simulink library "Library_SignalGeneration"  (R2017b)
settings: Solver=ode45  StartTime=0.0  StopTime=10.0  RelTol=1e-3  EnableMultiTasking=on
undefined symbols (not defined in the file): DiscIntNeverNeededParam, Fif, Fs, jsin, Ts
libraries: simulink x8, Library_SignalGeneration x5, simulink_need_slupdate x1
settings Model: Creator=Keith  LastModifiedBy=sawmilkd
settings DataIOCC: LimitDataPoints=on
settings OptimizationCC: LifeSpan=inf
settings DebuggingCC: AllowSymbolicDim=off  SFUnexpectedBacktrackingDiag=warning  SFNoUnconditionalDefaultTransitionDiag=warning  SFExecutionAtInitializationDiag=none
settings CodeAppCC: StateflowObjectComments=on
settings GRTTargetCC: TargetLangStandard=C89/C90 (ANSI)  GeneratePreprocessorConditionals=Disable all
settings ConfigComp: CovMetricSettings=dw  CovHtmlReporting=on  CovSaveCumulativeToWorkspaceVar=on  CovSaveSingleToWorkspaceVar=on  CovExternalEMLEnable=off

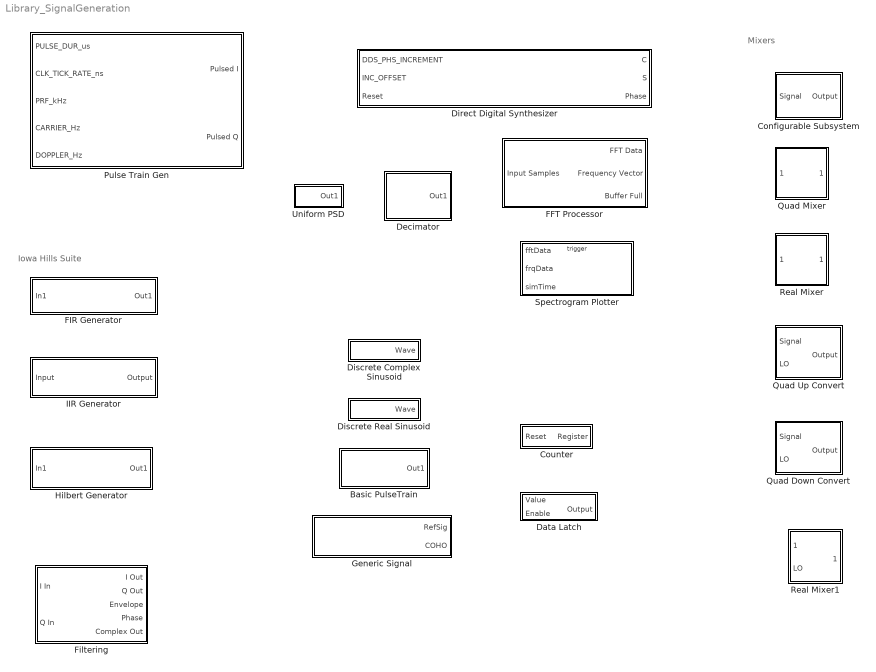
== system Library_SignalGeneration ==
  note: Iowa Hills Suite
  note: Mixers
  Basic PulseTrain : Subsystem  mask{Fs=245.76e6, PRF=633000, Fc=50e6, PD=0.6}
      mask prompts: Fs "Clock Rate"; PRF "PRF (Hz)"; Fc "Carrier (Hz)"; PD "Pulsewidth (us)"
      mask init:
      | iprf = floor(Fs/PRF)
      | ipd = floor(Fs*PD*1e-6)
      mask DialogControl DescTextVar Prompt: Generates clock-matched pulsetrain. This is the simplest form of pulsetrain generation.
      mask Display:
      | port_label('output',1,'')
      | disp([ ...
      |     'PRF: ' num2str(PRF) ' Hz\n' ...
      |     'PD: ' num2str(PD) ' us\n' ...
      |     'Fc: ' num2str(Fc/1e6) ' MHz' ...
      |     ]);
  Configurable Subsystem : Subsystem  BlockChoice=Quad Mixer
      settings: TemplateBlock=self  MemberBlocks=Quad Mixer,Real Mixer
  Counter : Subsystem  mask{nBits=0}
      mask prompts: nBits "Bits"
      mask Display:
      | nb = str2num(get_param(gcb,'nBits'));
      | if(nb == 0)
      |     disp(['CTR']);
      | 
      | else
      |     disp(['CTR' num2str(nb,'%d')]);
      | end
      | port_label('input',1,'R');
      | port_label('output',1,'O');
  Data Latch : Subsystem
  Decimator : Subsystem  mask{parentFs=Fs, decFac=2}
      mask prompts: parentFs "Parent Sample Rate"; decFac "Decimation Factor"
      mask DialogControl Control2 Prompt: Minimum Decimation is 2
      mask Display:
      | FD=parentFs/decFac;
      | str = 'Hz';
      | if(FD > 1e6)
      |     FD = FD/1e6;
      |     str = 'MHz';
      | elseif(FD > 1e3);
      |     FD = FD/1e3;
      |     str = 'kHz';
      | end
      | disp([num2str(decFac) ':1\nFD = ' num2str(FD) str])
  Direct Digital Synthesizer : Subsystem  mask{Fs=245.76e6, Nbits=28, useFreqInput=on}
      mask prompts: Fs "Clock Speed (Hz)"; Nbits "Bits"; useFreqInput "Frequency Based Input"
      mask DialogControl Control2 Prompt: This block can be configured to accept either integer phase increment and offsets or frequency (Hz) as an input
      mask Display:
      | if(useFreqInput)
      |     port_label('input',1,'F_Hz');
      |     port_label('input',2,'FO_Hz');
      | else
      |     port_label('input',1,'DDS_PHASE_INCREMENT')
      |     port_label('input',2,'DDS_PHASE_INC_OFFSET');
      | end
      | port_label('input',3,'Rst');
      | 
      | port_label('output',1,'Cos');
      | port_label('output',2,'Sin');
      | port_label('output',3,'Phase');
      | 
      | fprintf('Fs = %6.2fMHz\nBits = %d',Fs/1e6,Nbits);
  Discrete Complex Sinusoid : Subsystem  mask{initPhase=0*pi/180, freqHz=1e6-2000}
      mask prompts: initPhase "Starting Phase (rad)"; freqHz "Frequency (Hz)"
      settings: AttributesFormatString=|
      | Frequency: %<freqHz>
      | Starting Phase: %<initPhase>
  Discrete Real Sinusoid : Subsystem  mask{freqHz=5e6}
      mask prompts: freqHz "Frequency (Hz)"
      settings: AttributesFormatString=Frequency: %<freqHz>
  FFT Processor : Subsystem  mask{BUFFSIZE=2^10, FFTSIZE=2^10, FOUTRNG=[15 30]*1e6, OVLP_PRCNT=95, Fs=Fs, FSCALE=1e-6}
      mask prompts: BUFFSIZE "Buffer Size"; FFTSIZE "FFT Size"; FOUTRNG "Output Freq Range"; OVLP_PRCNT "% Overlap"; Fs "Input Rate"; FSCALE "Frequency Output Scale Factor"
      mask init:
      | %if(BUFFSIZE > FFTSIZE)
      | %    errordlg(['Buffer size (' num2str(BUFFSIZE) ') cannot exceed FFT size (' num2str(FFTSIZE) ').']);
      | %    BUFFSIZE = FFTSIZE;
      | %end
      | OVLP_FRAMES = floor((1-OVLP_PRCNT/100) * BUFFSIZE);
      | disp(['Overlap Frames: ' num2str(OVLP_FRAMES)]);
      | 
      | RateOut = Fs / BUFFSIZE;
      | DF = Fs / FFTSIZE;
      | 
      | 
      | 
      | if(isempty(FOUTRNG))
      |     FFTIDX = 1:FFTSIZE;
      | else
      |     spn = floor((FOUTRNG./Fs)*FFTSIZE);
      |     FFTIDX = spn(1):spn(2);
      | end
      | 
      | FFT_SIZE_OUT = length(FFTIDX);
      mask DialogControl Control2 Prompt: Buffer Size determines how many samples are accumulated before computing the FFT
      mask DialogControl Control3 Prompt: FFT Size determines how many samples (actual + zero padded) are passed to the FFT algorithm.
      mask DialogControl Control4 Prompt: Select the [fmin fmax] desired out of the FFT processor, or leave as [] to get the full spectrum.
      mask DialogControl Container3 Prompt: Information
      mask Display:
      | TimeOut = 1/RateOut;
      | if( TimeOut < 1.0e-3 )
      |     sf = 1.0e6;
      |     str = 'us';
      | elseif( TimeOut < 1.0e-0 )
      |     sf = 1000;
      |     str = 'ms';
      | else
      |     sf = 1;
      |     str = 's';
      | end
      | 
      | disp(['FO: ' num2str(RateOut) ' Hz'...
      |     '\nDF: ' num2str(DF) ' Hz' ...
      |     '\nDT: ' num2str(sf*TimeOut) str]);
      | port_label('input',1,'In');
      | port_label('output',1,'FFT');
      | port_label('output',2,'FRQ');
      | port_label('output',3,'FULL');
  FIR Generator : Subsystem  mask{ihFilename=<not specified>, ihFilenameResolved=<not specified>, fileIsVar=off, shiftEnable=off, shiftFactor=.3}
      mask prompts: ihFilename "Iowa Hills FIR Coefficient File"; fileIsVar "Filename above is a variable"; shiftEnable "Enable Quadrature Shifting"; shiftFactor "Shift Ratio (fraction of Fs)"
      mask init:
      | % Note: You can "access" dialog data directly, but to change
      | %       it, use the set_param command.
      | 
      | % Manage the dialog data. It can be:
      | % 1 - A filename, or 2 - A variable that evaluates to 
      | %     a filename.
      | 
      | % first, check for iowa hills code
      | s = which('FirFilterC');
      | if(isempty(s))
      |     errordlg('Iowa Hills not found in search path!','Iowa Hills Error');
      |     return;
      | end
      | 
      | 
      | instr = [];
      | if(~fileIsVar && ~strcmpi(ihFilename,'<not specified>'))
      |     instr = ihFilename;
      | elseif(fileIsVar && ~strcmpi(ihFilename,'<not specified>'))
      |     try
      |         instr = eval(ihFilename);
      |     catch
      |         instr = evalin('base',ihFilename);
      |     end
      | end
      | 
      | % Create MATLAB instance
      | if(~isempty(instr))
      |     set_param(gcb,'ihFilenameResolved',instr);
      |     
      |     if(~exist(instr,'file'))
      |         errordlg(['Could not locate file ' instr],'File Error');
      |         return;
      |     end
      |     
      |     local_instance = FirFilterC(instr);
      |     
      |     if(shiftEnable == 1)
      |         local_instance.shiftFir(shiftFactor,1);    
      |     end
      |     
      |     this_model = gcb;
      |     tgt_model = [this_model '/Discrete FIR Filter'];
      |     set_param(tgt_model,'Coefficients',['[' num2str(local_instance.tapgains.','%18.14f') ']']);
      | else
      |     set_param(gcb,'ihFilenameResolved','<not specified>');
      | end
      settings: AttributesFormatString=|
      | FIR File:  %<ihFilenameResolved>
      | Quad Shift: %<shiftEnable>,%<shiftFactor>
      mask DialogControl DescTextVar Prompt: Use the Iowa Hills Tools to develop the filter. You may either type the filename below, or store the filename as a variable and check the box below. In that case, enter the variable name in the field.
      mask DialogControl Control2 Prompt: The filter definition above may be shifted in frequency via quadrature shifting. This will create complex weights, but enables full spectrum IQ filtering
      mask Display:
      | s = get_param(gcb,'ihFilename');
      | if(strcmpi(s,'<not specified>'))
      |     fprintf('Iowa Hills FIR Filter\n %s',s);
      | else
      |     NFFT = 8192;
      |     xi = 0:NFFT-1;
      |     yi = str2num(get_param([gcb '/Discrete FIR Filter'],'Coefficients'));
      |     color('red');
      |     plot(xi,20*log10(abs(fft(yi,NFFT))));
      | end
  Filtering : Subsystem  mask{ihFirFile=BPF_50MHZ_245p76MGZ.txt}
      mask prompts: ihFirFile "Iowa Hills FIR Filter File"
      settings: AttributesFormatString=File: %<ihFirFile>
  Generic Signal : Subsystem  mask{fPoints=[0 0]*1e6 + Fif, dPoints=[20 24]*1e3, tPoints=[0 40*24e-3], isPulsed=on, PRF=600e3, PD=.5e-6, FS=Fs}
      mask prompts: fPoints "COHO Points"; dPoints "Doppler Points"; tPoints "Time Points"; isPulsed "Is Pulsed"; PD "Pulsewidth"
      mask init:
      | if(isPulsed)
      |     ipri = floor(FS/PRF);
      |     ipd = floor(FS * PD);
      | else
      |     ipri = 1;
      |     ipd = 1;
      | end
      | 
      | %disp([ipri ipd])
      mask Callback isPulsed:
      | if(strcmp('on',get_param(gcb,'isPulsed')))
      |     me = get_param(gcb,'MaskEnables');
      |     me{5} = 'on';
      |     me{6} = 'on';
      |     me{7} = 'on';
      | else
      |     me = get_param(gcb,'MaskEnables');
      |     me{5} = 'off';
      |     me{6} = 'off';
      |     me{7} = 'off';
      | end
      | set_param(gcb,'MaskEnables',me);
      mask DialogControl DescTextVar Prompt: Generates a reference quadrature signal with frequency properties specified over time
      mask DialogControl Control2 Prompt: COHO is Output CW, Doppler is not
      mask Display:
      | port_label('output',1,'SIG')
      | port_label('output',2,'COHO')
      | 
      | if(fPoints(1) > 1e6)
      |     fsc = 1e-6;
      |     fstr = 'MHz';
      | elseif(fPoints(1) > 1e3)
      |     fsc = 1e-3;
      |     fstr = 'kHz';
      | else
      |     fsc = 1.0;
      |     fstr = 'Hz';
      | end
      | 
      | if(PRF > 1e3)
      |     prfsc = 1e-3;
      |     prfstr = 'kHz';
      | else
      |     prfsc = 1.0;
      |     prfstr = 'Hz';
      | end
      | 
      | if(PD > 1e-3)
      |     pdsc = 1e3;
      |     pdstr = 'ms';
      | elseif(PD > 1e-6)
      |     pdsc = 1e6;
      |     pdstr = 'us';
      | elseif(PD > 1e-9)
      |     pdsc = 1e9;
      |     pdstr = 'ns';
      | end
      | 
      | 
      | if(isPulsed)
      |     text(0.15,.5,sprintf('F1=%4.2f%s\nPRF=%4.2f%s\nPW=%4.2f%s', ...
      |         fsc * fPoints(1),fstr,prfsc*PRF,prfstr,pdsc*PD,pdstr))
      | else
      |     text(0.15,.5,sprintf('F1=%4.2eHz\n\n',fPoints(1)))
      | end
  Hilbert Generator : Subsystem  mask{ihFilename=<not specified>, fileIsVar=off, ihFilenameResolved=<not specified>}
      mask prompts: ihFilename "Iowa Hills Hilbert Coefficient File"; fileIsVar "Filename above is a variable"
      mask init:
      | % Manage the dialog data. It can be:
      | % 1 - A filename, or 2 - A variable that evaluates to 
      | %     a filename.
      | instr = [];
      | if(~fileIsVar && ~strcmpi(ihFilename,'<not specified>'))
      |     instr = ihFilename;
      | elseif(fileIsVar && ~strcmpi(ihFilename,'<not specified>'))
      |     try
      |         instr = eval(ihFilename);
      |     catch
      |         instr = evalin('base',ihFilename);
      |     end
      | end
      | 
      | % Create MATLAB instance
      | if(~isempty(instr))
      |     set_param(gcb,'ihFilenameResolved',instr);
      |     local_instance = HilbertFilter(instr);
      |     this_model = gcb;
      |     tgt_model = [this_model '/Discrete FIR FilterI'];
      |     set_param(tgt_model,'Coefficients',['[' num2str(local_instance.iChanFIR.tapgains.','%18.14f') ']']);
      |     tgt_model = [this_model '/Discrete FIR FilterQ'];
      |     set_param(tgt_model,'Coefficients',['[' num2str(local_instance.qChanFIR.tapgains.','%18.14f') ']']);
      | else
      |     set_param(gcb,'ihFilenameResolved','<not specified>');
      | end
      settings: AttributesFormatString="Hilbert File:  %<ihFilenameResolved>"
      mask DialogControl DescTextVar Prompt: Use the Iowa Hills Tools to develop the filter. You may either type the filename below, or store the filename as a variable and check the box below. In that case, enter the variable name in the field.
      mask Display:
      | s = get_param(gcb,'ihFilename');
      | if(strcmpi(s,'<not specified>'))
      |     fprintf('Iowa Hills Hilbert Filter\n %s',s);
      | else
      |     NFFT = 8192;
      |     xi = 0:NFFT-1;
      |     yi = str2num(get_param([gcb '/Discrete FIR FilterQ'],'Coefficients'));
      |     color('red');
      |     plot(xi,20*log10(abs(fft(yi,NFFT))));
      | end
  IIR Generator : Subsystem  mask{ihFilename=<not specified>, shiftEnable=off, shiftFactor=0.5, bodeplt=0}
      mask prompts: ihFilename "Iowa Hills IIR Coefficient File"; shiftEnable "Enable Quadrature Shifting"; shiftFactor "Shift Ratio (fraction of Fs)"
      mask init:
      | %disp('Running IIR Init Mask Function')
      | 
      | % attempt to build IIR stages block via program
      | 
      | % first, read the file from MATLAB IH code
      | %disp([' Input Name: ' ihFilename]);
      | 
      | if(strcmp(ihFilename,'<not specified>'))
      |     return;
      | end
      | 
      | iir_file = ihFilename;
      | 
      | if(~exist(iir_file,'file'))
      |     errordlg(['Could not locate file ' iir_file],'File Error');
      |     return;
      | end
      | 
      | % Read in data
      | %local_instance = biquad_stages(0);
      | s = which('biquad_stages');
      | if(~isempty(s))
      |     local_instance = biquad_stages(iir_file);
      | else
      |     errordlg('Iowa Hills not found in search path!','Iowa Hills Error');
      |     return;
      | end
      | if(shiftEnable == 1)
      |    local_instance = local_instance.shiftStages(shiftFactor,1);    
      | end
      | npts=8192;
      | da = 2*pi*(0:npts)./npts;
      | z  = exp(1i*da);
      | bodeplt = 20*log10(abs(evalFilterZ(local_instance,z)));
      | %[a0,a1,a2,b0,b1,b2] = read_iowa_hills(iir_file);
      | 
      | src_model = gcb;
      | %disp([' Source model: ' src_model]);
      | 
      | % Prep model for building
      | h_lines = get_param(src_model,'Lines');
      | if(~isempty(h_lines))
      |     delete(h_lines(:).Handle);
      | end
      | 
      | h_blocks = get_param(src_model,'Blocks');
      | 
      | for k = 1 : length(h_blocks)
      |     if(strfind(h_blocks{k},'Stage'))
      |         %disp(['  Deleting existing block ' h_blocks{k}]);
      |         delete_block([src_model '/' h_blocks{k}])
      |     end
      | end
      | 
      | 
      | % spacing parameters
      | p_xstart = 70;
      | p_xoffset = 80;
      | 
      | nStages = local_instance.nstages;
      | %return;
      | %open_system(src_model);
      | 
      | dest_block_in = [src_model '/Input'];
      | %add_block( ...
      | %    'simulink/Sources/In1', ...
      | %    dest_block_in);
      | set_param(dest_block_in,'Position', ...
      |     [0+p_xstart 38 0+30+p_xstart 52]);
      | 
      | 
      | for istage = 1 :nStages
      |     dest_block = [src_model '/Stage ' num2str(istage-1)];
      |     add_block( ...
      |         'simulink/Discrete/Discrete Filter', ...
      |         dest_block);
      |     
      |     % NOTE: Position is topleft x,y, botright x,y
      |     xoffset = p_xoffset*(istage);
      |     xstart = p_xstart;
      |     set_param(dest_block,'Position',[xstart+xoffset 25 xstart+50+xoffset 60]);
      |     
      |     % set the connection to blocks
      |     if(istage == 1)
      |         add_line(src_model,'Input/1','Stage 0/1');
      |     else
      |         add_line(src_model, ...
      |             ['Stage ' num2str(istage-2) '/1'], ...
      |             ['Stage ' num2str(istage-1) '/1']);
      |     end
      |     
      |     % evaluate shifting
      |     %disp(shiftEnable)
      | %     if(shiftEnable == 1)
      | %          k = 1; sc1 = exp(1i*2*pi*shiftFactor*k);
      | %          k = 2; sc2 = exp(1i*2*pi*shiftFactor*k);
      | %     else
      | %         sc1 = 1;
      | %         sc2 = 1;
      | %     end
      |     
      |     
      |     % set the coefficients
      |     %str = ['[' num2str([a0(istage) sc1*a1(istage) sc2*a2(istage)],'%18.14f ') ']'];
      |     str = ['[' num2str(local_instance.biquads(istage).A,'%18.14f') ']'];
      |     set_param(dest_block,'Denominator',str);
      |     %str = ['[' num2str([b0(istage) sc1*b1(istage) sc2*b2(istage)],'%18.14f ') ']'];
      |     str = ['[' num2str(local_instance.biquads(istage).B,'%18.14f') ']'];
      |     set_param(dest_block,'Numerator',str);
      |     set_param(dest_block,'SampleTime','-1');
      |     
      | end
      | 
      | dest_block_out = [src_model '/Output'];
      | %add_block( ...
      | %    'simulink/Sinks/Out1', ...
      | %    dest_block_out);
      | xoffset = p_xoffset*(istage+1);
      | set_param(dest_block_out,'Position', ...
      |     [0+p_xstart+xoffset 38 0+30+p_xstart+xoffset 52]);
      | 
      | add_line(src_model, ...
      |         ['Stage ' num2str(istage-1) '/1'], ...
      |         ['Output/1']);
      settings: AttributesFormatString=|
      | IIR File:  %<ihFilename>
      | Quad Shift: %<shiftEnable>,%<shiftFactor>
      mask DialogControl Control2 Prompt: The filter definition above may be shifted in frequency via quadrature shifting. This will create complex weights, but enables full spectrum IQ filtering
      mask Display:
      | s = get_param(gcb,'ihFilename');
      | if(strcmpi(s,'<not specified>'))
      |     fprintf('Iowa Hills IIR Filter\n %s',s);
      | else
      |     plot(bodeplt);
      | end
  Pulse Train Gen : Subsystem
  Quad Down Convert : Subsystem
      mask Display: image('mixer_3port.png');
  Quad Mixer : Subsystem  mask{loFrequencyHz=-4e6}
      mask prompts: loFrequencyHz "LO Frequency (Hz)"
      settings: AttributesFormatString=LO: %<loFrequencyHz>
      mask DialogControl DescTextVar Prompt: This block will take a complex input and either upconvert (+) or downconvert (-) by the mixing with a complex specified LO (below)
      mask Display:
      | image('mixer2.png');
      | %port_label('output', 1, 'O')
      | %port_label('input', 1, 'I')
  Quad Up Convert : Subsystem
      mask Display: image('mixer_3port.png');
  Real Mixer : Subsystem  mask{loFrequencyHz=-4e6}
      mask prompts: loFrequencyHz "LO Frequency (Hz)"
      settings: AttributesFormatString=LO: %<loFrequencyHz>
      mask DialogControl DescTextVar Prompt: This block will take a complex input and either upconvert (+) or downconvert (-) by the mixing with a complex specified LO (below)
      mask Display:
      | image('mixer2.png');
      | %port_label('output', 1, 'O')
      | %port_label('input', 1, 'I')
  Real Mixer1 : Subsystem  mask{loFrequencyHz=-4e6}
      mask prompts: loFrequencyHz "LO Frequency (Hz)"
      settings: AttributesFormatString=LO: %<loFrequencyHz>
      mask DialogControl DescTextVar Prompt: This block will take a complex input and either upconvert (+) or downconvert (-) by the mixing with a complex specified LO (below)
      mask Display:
      | %image('mixer2.png');
      | port_label('output', 1, 'IF')
      | port_label('input', 2, 'RF')
      | port_label('input', 1, 'LO')
  Spectrogram Plotter : MATLAB Function  StopFcn=disp('done')  TreatAsAtomicUnit=on  mask{nRows=64, complexFFT=on, Fs=1000, Zo=50, cMin=-60, cMax=10}
      mask prompts: nRows "Rows in Image"; complexFFT "Quadrature Data? (Use Fs vs Fs/2)"; Fs "Sample Rate (Hz)"; Zo "Characteristic Impedance (Ohms)"; cMin "Minimum Power Scale"; cMax "Maximum Power Scale"
      settings: AttributesFormatString=|
      | Fs=%<Fs> | Zo=%<Zo>
      | Displays %<nRows> Rows
  Uniform PSD : Subsystem  mask{nzdb=4.5, reftemp=290, Fs=245.76e6}
      mask prompts: nzdb "Noise Figure (dB)"; reftemp "Reference Temp (K)"; Fs "Fs (Hz)"
      mask Display: disp([get_param(gcb,'nzdb') 'dB'])

== system Library_SignalGeneration/Basic PulseTrain ==
  Discrete Complex Sinusoid : Library_SignalGeneration/Discrete Complex Sinusoid  freqHz=Fc
      settings: AttributesFormatString=Frequency: %<freqHz>
  Product : Product
  Pulse Generator : DiscretePulseGenerator  Period=iprf  PulseWidth=ipd  SampleTime=Ts
  Out1 : Outport
  wires:
  Discrete Complex Sinusoid/1 -> Product/1
  Pulse Generator/1 -> Product/2
  Product/1 -> Out1/1

== system Library_SignalGeneration/Configurable Subsystem ==
  Signal : Inport
  Quad Mixer : Library_SignalGeneration/Quad Mixer  loFrequencyHz=-4e6
      settings: AttributesFormatString=LO: %<loFrequencyHz>
  Output : Outport
  wires:
  Signal/1 -> Quad Mixer/1
  Quad Mixer/1 -> Output/1

== system Library_SignalGeneration/Counter ==
  note: Increments when reset pin is low, resets on pin == 1
  Reset : Inport
  MATLAB Function : MATLAB Function  TreatAsAtomicUnit=on
  Unit Delay : UnitDelay  InitialCondition=-1  SampleTime=-1
  Register : Outport
  wires:
  MATLAB Function/1(y) -> Unit Delay/1, Register/1
  Reset/1 -> MATLAB Function/2(reset)
  Unit Delay/1 -> MATLAB Function/1(u)

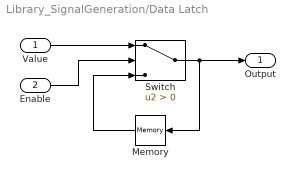
== system Library_SignalGeneration/Data Latch ==
  Value : Inport
  Enable : Inport  Port=2
  Memory : Memory
  Switch : Switch  Criteria=u2 > Threshold
  Output : Outport
  wires:
  Enable/1 -> Switch/2
  Value/1 -> Switch/1
  Switch/1 -> Output/1, Memory/1
  Memory/1 -> Switch/3

== system Library_SignalGeneration/Decimator ==
  Compare To Constant1 : simulink/Logic and Bit Operations/Compare To Constant  relop===  const=decFac-1  OutDataTypeStr=boolean
  Counter Limited : simulink/Sources/Counter Limited  uplimit=decFac-1  tsamp=-1
  Scope : Scope  NumInputPorts=2
  Out1 : Outport
  wires:
  Compare To Constant1/1 -> Out1/1, Scope/2
  Counter Limited/1 -> Compare To Constant1/1, Scope/1

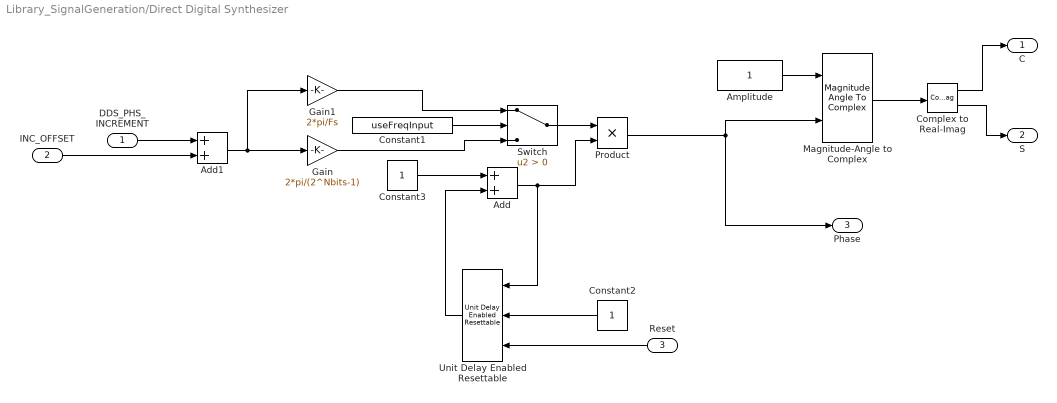
== system Library_SignalGeneration/Direct Digital Synthesizer ==
  DDS_PHS_INCREMENT : Inport
  INC_OFFSET : Inport  Port=2
  Reset : Inport  Port=3
  Add : Sum
  Add1 : Sum
  Amplitude : Constant
  Complex to Real-Imag : ComplexToRealImag
  Constant1 : Constant  Value=useFreqInput
  Constant2 : Constant
  Constant3 : Constant
  Gain : Gain  Gain=2*pi/(2^Nbits-1)
  Gain1 : Gain  Gain=2*pi/Fs
  Magnitude-Angle to Complex : MagnitudeAngleToComplex
  Product : Product
  Switch : Switch  Criteria=u2 > Threshold
  Unit Delay Enabled Resettable : simulink_need_slupdate/Unit Delay Enabled Resettable  vinit=1  tsamp=-1
      settings: SourceProductName=Simulink  SourceProductBaseCode=SL
  C : Outport
  S : Outport  Port=2
  Phase : Outport  Port=3
  wires:
  Gain1/1 -> Switch/1
  Gain/1 -> Switch/3
  Amplitude/1 -> Magnitude-Angle to Complex/1
  Product/1 -> Phase/1, Magnitude-Angle to Complex/2
  Unit Delay Enabled Resettable/1 -> Add/2
  Constant2/1 -> Unit Delay Enabled Resettable/2
  Add/1 -> Unit Delay Enabled Resettable/1, Product/2
  Constant3/1 -> Add/1
  Add1/1 -> Gain/1, Gain1/1
  Magnitude-Angle to Complex/1 -> Complex to Real-Imag/1
  DDS_PHS_INCREMENT/1 -> Add1/1
  Reset/1 -> Unit Delay Enabled Resettable/3
  Complex to Real-Imag/1 -> C/1
  Complex to Real-Imag/2 -> S/1
  INC_OFFSET/1 -> Add1/2
  Switch/1 -> Product/1
  Constant1/1 -> Switch/2

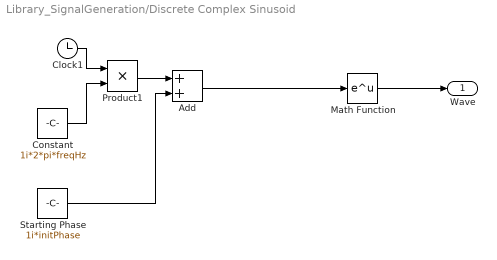
== system Library_SignalGeneration/Discrete Complex Sinusoid ==
  Add : Sum
  Clock1 : Clock
  Constant : Constant  Value=1i*2*pi*freqHz
  Math Function : Math  OutputSignalType=complex  SaturateOnIntegerOverflow=on
  Product1 : Product
  Starting Phase : Constant  Value=1i*initPhase
  Wave : Outport
  wires:
  Add/1 -> Math Function/1
  Starting Phase/1 -> Add/2
  Product1/1 -> Add/1
  Math Function/1 -> Wave/1
  Clock1/1 -> Product1/1
  Constant/1 -> Product1/2

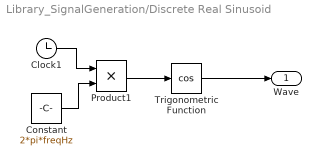
== system Library_SignalGeneration/Discrete Real Sinusoid ==
  Clock1 : Clock
  Constant : Constant  Value=2*pi*freqHz
  Product1 : Product
  Trigonometric Function : Trigonometry  Operator=cos
  Wave : Outport
  wires:
  Product1/1 -> Trigonometric Function/1
  Constant/1 -> Product1/2
  Clock1/1 -> Product1/1
  Trigonometric Function/1 -> Wave/1

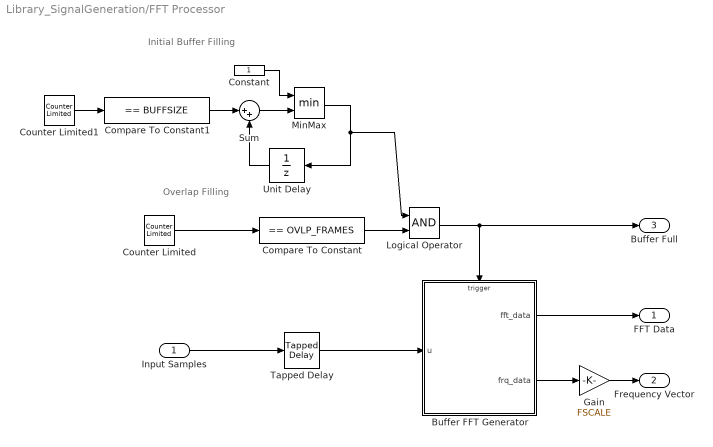
== system Library_SignalGeneration/FFT Processor ==
  note: Overlap Filling
  note: Initial Buffer Filling
  Input Samples : Inport
  Buffer FFT Generator : MATLAB Function  TreatAsAtomicUnit=on  mask{NFFT=FFTSIZE, NBUF=BUFFSIZE, FFTIDX=FFTIDX}
      mask prompts: NFFT "# of FFT Points?"; NBUF "Input Buffer Size?"; FFTIDX "FFT Output Bins"
      settings: AttributesFormatString=|
      | Buffer Size:%<NBUF>
      | FFT Size:%<NFFT>
  Compare To Constant : simulink/Logic and Bit Operations/Compare To Constant  relop===  const=OVLP_FRAMES  OutDataTypeStr=boolean
  Compare To Constant1 : simulink/Logic and Bit Operations/Compare To Constant  relop===  const=BUFFSIZE  OutDataTypeStr=uint8
  Constant : Constant  OutDataTypeStr=uint8
  Counter Limited : simulink/Sources/Counter Limited  uplimit=OVLP_FRAMES  tsamp=-1
  Counter Limited1 : simulink/Sources/Counter Limited  uplimit=BUFFSIZE  tsamp=-1
  Gain : Gain  Gain=FSCALE
  Logical Operator : Logic  AllPortsSameDT=off  OutDataTypeStr=boolean
  MinMax : MinMax  Inputs=2
  Sum : Sum  Inputs=|++
  Tapped Delay : simulink/Discrete/Tapped Delay  vinit=0  samptime=-1  NumDelays=BUFFSIZE-1  DelayOrder=Oldest  includeCurrent=on
  Unit Delay : UnitDelay  SampleTime=-1
  FFT Data : Outport
  Frequency Vector : Outport  Port=2
  Buffer Full : Outport  Port=3
  wires:
  Input Samples/1 -> Tapped Delay/1
  Tapped Delay/1 -> Buffer FFT Generator/1(u)
  Counter Limited/1 -> Compare To Constant/1
  Buffer FFT Generator/1(fft_data) -> FFT Data/1
  Buffer FFT Generator/2(frq_data) -> Gain/1
  Counter Limited1/1 -> Compare To Constant1/1
  Sum/1 -> MinMax/2
  Compare To Constant1/1 -> Sum/1
  Unit Delay/1 -> Sum/2
  MinMax/1 -> Unit Delay/1, Logical Operator/1
  Constant/1 -> MinMax/1
  Compare To Constant/1 -> Logical Operator/2
  Logical Operator/1 -> Buffer Full/1, Buffer FFT Generator/Trigger
  Gain/1 -> Frequency Vector/1

== system Library_SignalGeneration/FIR Generator ==
  In1 : Inport
  Discrete FIR Filter : DiscreteFir  Coefficients="[0.0026555053703067-0.0081728051610735i   0.0013074417466856+0.0009499120318567i   0.0069800854624918-0.0050713289376123i   0.0054570299903825+0.0167950113632718i  -0.0201941364377624+0.0000000000000000i   0.0039181695206914-0.0120588858296939i  -0.0035112262148963-0.0025510551705694i   0.0204105317318432-0.0148291193223870i   0.0124875056110475+0.0384325904395045i  -0.0395603457642835+0.0000000000000000i   0.0048748446363794-0.0150032290836721i  -0.0250312689023583-0.0181862813875014i   0.0747917324181241-0.0543393743449645i   0.0476754456218221+0.1467299341177754i  -0.2000561505185882+0.0000000000000009i   0.0670354126806467-0.2063137860149763i   0.1618488255987701+0.1175900549052298i  -0.1248159370667271+0.0906840864518182i  -0.0285678997062365-0.0879229546175564i   0.0309403499263914-0.0000000000000000i   0.0048748446363795-0.0150032290836721i   0.0320049920266545+0.0232529878158365i  -0.0326927141244272+0.0237526471673182i  -0.0077961293931059-0.0239940190868500i   0.0043401142859911+0.0000000000000000i   0.0039181695206914-0.0120588858296939i   0.0163373995648762+0.0118698155808987i  -0.0142866899924488+0.0103798878639427i  -0.0026661554022928-0.0082055825891876i  -0.0016160868755245+0.0000000000000000i   0.0026555053703067-0.0081728051610735i]"  InputProcessing=Columns as channels (frame based)
  Out1 : Outport
  wires:
  Discrete FIR Filter/1 -> Out1/1
  In1/1 -> Discrete FIR Filter/1

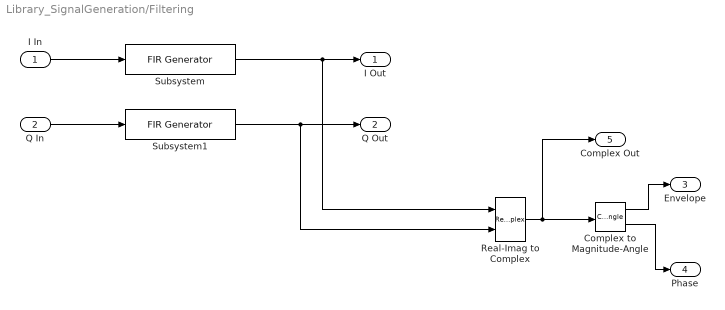
== system Library_SignalGeneration/Filtering ==
  I In : Inport
  Q In : Inport  Port=2
  Complex to Magnitude-Angle : ComplexToMagnitudeAngle
  Real-Imag to Complex : RealImagToComplex
  Subsystem : Library_SignalGeneration/FIR Generator  ihFilename=get_param(get_param(gcb,'Parent'),'ihFirFile')  ihFilenameResolved=BPF_50MHZ_245p76MGZ.txt  fileIsVar=on  shiftEnable=off  shiftFactor=.3
  Subsystem1 : Library_SignalGeneration/FIR Generator  ihFilename=get_param(get_param(gcb,'Parent'),'ihFirFile')  ihFilenameResolved=BPF_50MHZ_245p76MGZ.txt  fileIsVar=on  shiftEnable=off  shiftFactor=.3
  I Out : Outport
  Q Out : Outport  Port=2
  Envelope : Outport  Port=3
  Phase : Outport  Port=4
  Complex Out : Outport  Port=5
  wires:
  Subsystem1/1 -> Q Out/1, Real-Imag to Complex/2
  Subsystem/1 -> I Out/1, Real-Imag to Complex/1
  Q In/1 -> Subsystem1/1
  I In/1 -> Subsystem/1
  Complex to Magnitude-Angle/1 -> Envelope/1
  Complex to Magnitude-Angle/2 -> Phase/1
  Real-Imag to Complex/1 -> Complex to Magnitude-Angle/1, Complex Out/1

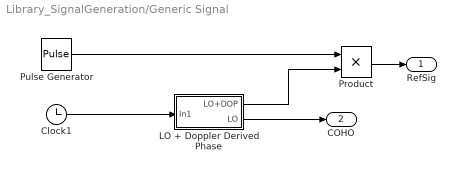
== system Library_SignalGeneration/Generic Signal ==
  Clock1 : Clock
  LO + Doppler Derived Phase : Subsystem
  Product : Product
  Pulse Generator : DiscretePulseGenerator  Period=ipri  PulseWidth=ipd  SampleTime=Ts
  RefSig : Outport
  COHO : Outport  Port=2
  wires:
  Clock1/1 -> LO + Doppler Derived Phase/1(In1)
  LO + Doppler Derived Phase/1(LO+DOP) -> Product/2
  Pulse Generator/1 -> Product/1
  Product/1 -> RefSig/1
  LO + Doppler Derived Phase/2(LO) -> COHO/1

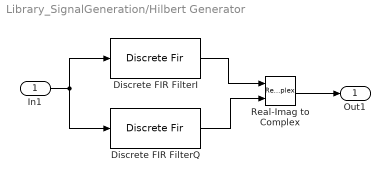
== system Library_SignalGeneration/Hilbert Generator ==
  In1 : Inport
  Discrete FIR FilterI : DiscreteFir  Coefficients=[]  InputProcessing=Columns as channels (frame based)
  Discrete FIR FilterQ : DiscreteFir  Coefficients=[]  InputProcessing=Columns as channels (frame based)
  Real-Imag to Complex : RealImagToComplex
  Out1 : Outport
  wires:
  In1/1 -> Discrete FIR FilterI/1, Discrete FIR FilterQ/1
  Discrete FIR FilterI/1 -> Real-Imag to Complex/1
  Discrete FIR FilterQ/1 -> Real-Imag to Complex/2
  Real-Imag to Complex/1 -> Out1/1

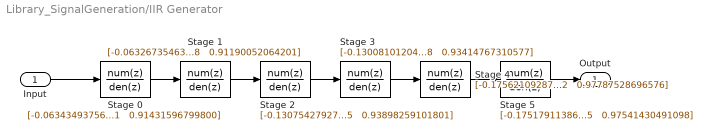
== system Library_SignalGeneration/IIR Generator ==
  Input : Inport
  Stage 0 : DiscreteFilter  Numerator="[-0.06343493756448   0.00000000000000   0.06343493756448]"  Denominator="[1.00000000000000  -0.63960783794761   0.91431596799800]"
  Stage 1 : DiscreteFilter  Numerator="[-0.06326735463081   0.00000000000000   0.06326735463081]"  Denominator="[1.00000000000000  -0.46230125035858   0.91190052064201]"
  Stage 2 : DiscreteFilter  Numerator="[-0.13075427927884   0.00000000000000   0.13075427927884]"  Denominator="[1.00000000000000  -0.79283413386325   0.93898259101801]"
  Stage 3 : DiscreteFilter  Numerator="[-0.13008101204999   0.00000000000000   0.13008101204999]"  Denominator="[1.00000000000000  -0.30659331922548   0.93414767310577]"
  Stage 4 : DiscreteFilter  Numerator="[-0.17562109287705   0.00000000000000   0.17562109287705]"  Denominator="[1.00000000000000  -0.88878765257452   0.97787528696576]"
  Stage 5 : DiscreteFilter  Numerator="[-0.17517911386012   0.00000000000000   0.17517911386012]"  Denominator="[1.00000000000000  -0.21689129681705   0.97541430491098]"
  Output : Outport
  wires:
  Input/1 -> Stage 0/1
  Stage 0/1 -> Stage 1/1
  Stage 1/1 -> Stage 2/1
  Stage 2/1 -> Stage 3/1
  Stage 3/1 -> Stage 4/1
  Stage 4/1 -> Stage 5/1
  Stage 5/1 -> Output/1

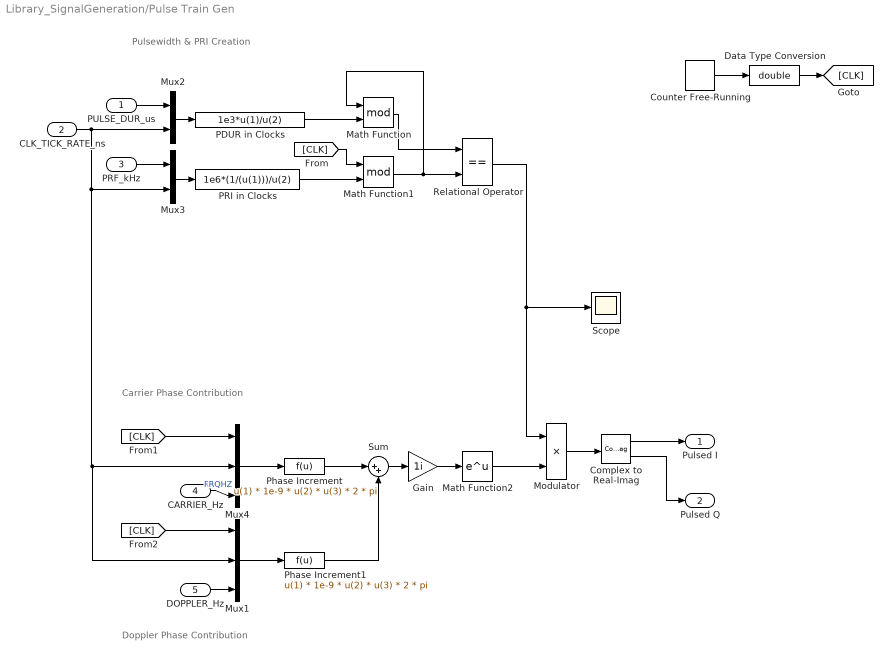
== system Library_SignalGeneration/Pulse Train Gen ==
  note: Pulsewidth & PRI Creation
  note: Doppler Phase Contribution
  note: Carrier Phase Contribution
  PULSE_DUR_us : Inport
  CLK_TICK_RATE_ns : Inport  Port=2
  PRF_kHz : Inport  Port=3
  CARRIER_Hz : Inport  Port=4
  DOPPLER_Hz : Inport  Port=5
  Complex to Real-Imag : ComplexToRealImag
  Counter Free-Running : simulink/Sources/Counter Free-Running  NumBits=64  tsamp=-1
  Data Type Conversion : DataTypeConversion  OutDataTypeStr=double
  Gain : Gain  Gain=1i
  Math Function : Math  Operator=mod  SaturateOnIntegerOverflow=on
  Math Function1 : Math  Operator=mod  SaturateOnIntegerOverflow=on
  Math Function2 : Math  SaturateOnIntegerOverflow=on
  Modulator : Product
  Mux1 : Mux  Inputs=3
  Mux2 : Mux  Inputs=2
  Mux3 : Mux  Inputs=2
  Mux4 : Mux  Inputs=3
  PDUR in Clocks : Fcn  Expr=1e3*u(1)/u(2)
  PRI in Clocks : Fcn  Expr=1e6*(1/(u(1)))/u(2)
  Phase Increment : Fcn  Expr=u(1) * 1e-9 * u(2) * u(3) * 2 * pi
  Phase Increment1 : Fcn  Expr=u(1) * 1e-9 * u(2) * u(3) * 2 * pi
  Relational Operator : RelationalOperator  Operator===  OutDataTypeStr=boolean  RndMeth=Nearest
  Scope : Scope
  Sum : Sum  Inputs=|++
  Pulsed I : Outport
  Pulsed Q : Outport  Port=2
  wires:
  Gain/1 -> Math Function2/1
  [CLK] -> Mux1/1
  Mux1/1 -> Phase Increment1/1
  DOPPLER_Hz/1 -> Mux1/3
  Phase Increment1/1 -> Sum/2
  Phase Increment/1 -> Sum/1
  Sum/1 -> Gain/1
  Math Function2/1 -> Modulator/2
  Complex to Real-Imag/2 -> Pulsed Q/1
  Complex to Real-Imag/1 -> Pulsed I/1
  Modulator/1 -> Complex to Real-Imag/1
  Relational Operator/1 -> Modulator/1, Scope/1
  [CLK] -> Mux4/1
  CARRIER_Hz/1 -> Mux4/3  "FRQHZ"
  Mux4/1 -> Phase Increment/1
  PDUR in Clocks/1 -> Math Function/2
  Math Function/1 -> Relational Operator/1
  Math Function1/1 -> Relational Operator/2, Math Function/1
  PRI in Clocks/1 -> Math Function1/2
  [CLK] -> Math Function1/1
  Data Type Conversion/1 -> [CLK]
  PRF_kHz/1 -> Mux3/1
  Mux3/1 -> PRI in Clocks/1
  Counter Free-Running/1 -> Data Type Conversion/1
  CLK_TICK_RATE_ns/1 -> Mux2/2, Mux3/2, Mux4/2, Mux1/2
  PULSE_DUR_us/1 -> Mux2/1
  Mux2/1 -> PDUR in Clocks/1

== system Library_SignalGeneration/Quad Down Convert ==
  Signal : Inport
  LO : Inport  Port=2
  Product : Product  Inputs=/*
  Output : Outport
  wires:
  Product/1 -> Output/1
  Signal/1 -> Product/2
  LO/1 -> Product/1

== system Library_SignalGeneration/Quad Mixer ==
  Signal : Inport
  Discrete Complex Sinusoid : Subsystem  mask{freqHz=loFrequencyHz}
      mask prompts: freqHz "Frequency (Hz)"
      settings: AttributesFormatString=Frequency: %<freqHz>
  Product : Product
  Output : Outport
  wires:
  Product/1 -> Output/1
  Signal/1 -> Product/2
  Discrete Complex Sinusoid/1(Wave) -> Product/1

== system Library_SignalGeneration/Quad Up Convert ==
  Signal : Inport
  LO : Inport  Port=2
  Product : Product
  Output : Outport
  wires:
  LO/1 -> Product/1
  Signal/1 -> Product/2
  Product/1 -> Output/1

== system Library_SignalGeneration/Real Mixer ==
  Signal : Inport
  Discrete Real Sinusoid : Library_SignalGeneration/Discrete Real Sinusoid  freqHz=loFrequencyHz
      settings: AttributesFormatString=Frequency: %<freqHz>
  Product : Product
  Output : Outport
  wires:
  Product/1 -> Output/1
  Signal/1 -> Product/2
  Discrete Real Sinusoid/1 -> Product/1

== system Library_SignalGeneration/Real Mixer1 ==
  Signal : Inport
  LO : Inport  Port=2
  Product : Product
  Output : Outport
  wires:
  Signal/1 -> Product/2
  Product/1 -> Output/1
  LO/1 -> Product/1

== system Library_SignalGeneration/Uniform PSD ==
  Gain : Gain  Gain=1i
  Gain1 : Gain  Gain=sqrt(10^(0.1*nzdb)*1.38e-23*reftemp*Fs)
  Math Function : Math  OutputSignalType=complex  SaturateOnIntegerOverflow=on
  Uniform Random Number : UniformRandomNumber  Minimum=0  Maximum=2*pi
  Out1 : Outport
  wires:
  Gain1/1 -> Out1/1
  Uniform Random Number/1 -> Gain/1
  Gain/1 -> Math Function/1
  Math Function/1 -> Gain1/1

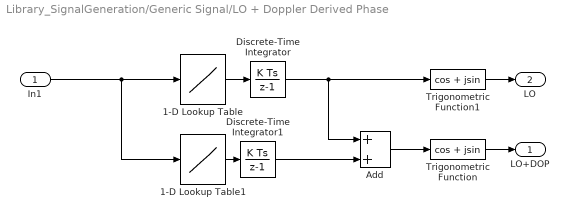
== system Library_SignalGeneration/Generic Signal/LO + Doppler Derived Phase ==
  In1 : Inport
  1-D Lookup Table : Lookup_n-D  NumberOfTableDimensions=1  BreakpointsForDimension1=tPoints  BeginIndexSearchUsingPreviousIndexResult=on  Table=fPoints  InternalRulePriority=Speed  RndMeth=Simplest  InputSameDT=on
  1-D Lookup Table1 : Lookup_n-D  NumberOfTableDimensions=1  BreakpointsForDimension1=tPoints  BeginIndexSearchUsingPreviousIndexResult=on  Table=dPoints  InternalRulePriority=Speed  RndMeth=Simplest  InputSameDT=on
  Add : Sum
  Discrete-Time Integrator : DiscreteIntegrator  gainval=2*pi  InitialConditionSetting=State (most efficient)  SampleTime=-1  ICPrevOutput=DiscIntNeverNeededParam  ICPrevScaledInput=DiscIntNeverNeededParam
  Discrete-Time Integrator1 : DiscreteIntegrator  gainval=2*pi  InitialConditionSetting=State (most efficient)  SampleTime=-1  ICPrevOutput=DiscIntNeverNeededParam  ICPrevScaledInput=DiscIntNeverNeededParam
  Trigonometric Function : Trigonometry  Operator=cos + jsin
  Trigonometric Function1 : Trigonometry  Operator=cos + jsin
  LO+DOP : Outport
  LO : Outport  Port=2
  wires:
  Trigonometric Function/1 -> LO+DOP/1
  1-D Lookup Table/1 -> Discrete-Time Integrator/1
  In1/1 -> 1-D Lookup Table1/1, 1-D Lookup Table/1
  1-D Lookup Table1/1 -> Discrete-Time Integrator1/1
  Discrete-Time Integrator1/1 -> Add/2
  Trigonometric Function1/1 -> LO/1
  Discrete-Time Integrator/1 -> Add/1, Trigonometric Function1/1
  Add/1 -> Trigonometric Function/1

== system Library_SignalGeneration/Quad Mixer/Discrete Complex Sinusoid ==
  Clock1 : Clock
  Constant : Constant  Value=1i*2*pi*freqHz
  Math Function : Math  SaturateOnIntegerOverflow=on
  Product1 : Product
  Wave : Outport
  wires:
  Product1/1 -> Math Function/1
  Constant/1 -> Product1/2
  Clock1/1 -> Product1/1
  Math Function/1 -> Wave/1

== matlab function Library_SignalGeneration/Spectrogram Plotter ==
  data: fftData input; frqData input; nRows parameter double; complexFFT parameter; Fs parameter; Zo parameter; cMin parameter; cMax parameter; simTime input
  events: trigger input RISING_EDGE_EVENT
function fcn(fftData,frqData, nRows, complexFFT, Fs, Zo, cMin, cMax, simTime)
coder.extrinsic('imagesc')
coder.extrinsic('colorbar')
coder.extrinsic('num2str')
coder.extrinsic('sprintf')

persistent imHandle
persistent cbHandle
persistent drawRow
persistent drawData
persistent indexToData
persistent frqVectorToUse
persistent normValue
persistent hT


if(isempty(drawRow)) % first time through it all
    if(complexFFT)
        indexToData = 1:length(frqData);
        drawData = zeros(nRows,length(indexToData));
        normValue = length(fftData);
    else
        indexToData = 1:floor(length(frqData)/2);
        drawData = zeros(nRows,length(indexToData))-300;
        normValue = floor(length(fftData)/2);
    end
    drawRow = 0;
    frqVectorToUse = Fs * frqData(indexToData);
    
end

if(drawRow < nRows)
    drawRow = drawRow + 1;
else
    drawData = drawData([2:end 1],:);
end

drawData(drawRow,:) = 20*log10(abs(fftData(indexToData))./normValue)-10*log10(2*Zo) + 30;



if(isempty(imHandle))
    figure;
    imHandle = imagesc(frqVectorToUse,1:nRows,drawData);
    %set(imHandle,'UserData',gcb);
    cbHandle = colorbar;
    %str1 = ['Power Spectrum (dBm), ];
    hT = title(['Power Spectrum (dBm), Time: ' num2str(simTime,'%18.12f')]);
    if(cMin ~= 0 || cMax ~= 0)
        set(cbHandle,'Limits',[cMin cMax]);
        caxis([cMin cMax]);
    end
    xlabel('Frequency');
    ylabel('Time');
else
    set(imHandle,'CData',drawData);
    set(hT,'String',['Power Spectrum (dBm), Time: ' num2str(simTime,'%18.12f')]);
end

drawnow;

== matlab function Library_SignalGeneration/FFT Processor/Buffer FFT Generator ==
  data: u input; fft_data output size=FFT_SIZE_OUT; frq_data output size=FFT_SIZE_OUT; NFFT parameter; NBUF parameter; FFTIDX parameter
  events: trigger input RISING_EDGE_EVENT
function [fft_data,frq_data] = fcn(u, NFFT, NBUF,FFTIDX)
%#codegen
temp = fft(u,NFFT);
fft_data = temp(FFTIDX);
temp = (0:NFFT-1)'/NFFT;
frq_data = temp(FFTIDX);

== matlab function Library_SignalGeneration/Counter/MATLAB Function ==
  data: u input; reset input; y output; nBits parameter
function y = fcn(u,reset,nBits)
if(reset)
    y = 0;
    return;
end
if((nBits ~= 0) && (u >= (2^(nBits)-1)))
    y = 0;
else
    y = u+1;
end
